simulink model "chap8_5sim"  (Simulink 7.7)
settings: Solver=ode45  StartTime=0.0  StopTime=10  RelTol=1e-3
settings Model: Creator=ljk  LastModifiedBy=ljk  ExtModeTrigMode=oneshot  ExtModeArmWhenConnect=off
settings DataIOCC: LimitDataPoints=off
settings OptimizationCC: BlockReduction=off  BooleanDataType=off
settings DebuggingCC: SaveWithParameterizedLinksMsg=none  SignalResolutionControl=TryResolveAllWithWarning  SolverPrmCheckMsg=none  MultiTaskDSMMsg=warning  MultiTaskCondExecSysMsg=none  StrictBusMsg=None
settings HardwareCC: TargetUnknown=on
settings RTWCC: IncludeERTFirstTime=on

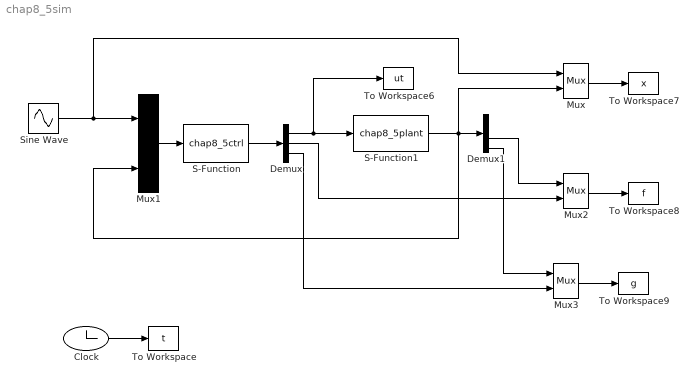
== system chap8_5sim ==
  Clock : Clock
  Demux : Demux  Outputs=3
  Demux1 : Demux
  Mux{,1..3} (4 alike) : Mux  Inputs=2
  S-Function : S-Function  FunctionName=chap8_5ctrl  EnableBusSupport=off
  S-Function1 : S-Function  FunctionName=chap8_5plant  EnableBusSupport=off
  Sine Wave : Sin  Amplitude=0.1  SampleTime=0
  To Workspace : ToWorkspace  VariableName=t  SampleTime=-1  SaveFormat=Array
  To Workspace6 : ToWorkspace  VariableName=ut  SampleTime=-1  SaveFormat=Array
  To Workspace7 : ToWorkspace  VariableName=x  SampleTime=-1  SaveFormat=Array
  To Workspace8 : ToWorkspace  VariableName=f  SampleTime=-1  SaveFormat=Array
  To Workspace9 : ToWorkspace  VariableName=g  SampleTime=-1  SaveFormat=Array
  wires:
  Mux1/1 -> S-Function/1
  S-Function/1 -> Demux/1
  S-Function1/1 -> Demux1/1, Mux/2, Mux1/2
  Sine Wave/1 -> Mux/1, Mux1/1
  Demux/3 -> Mux3/2
  Demux/2 -> Mux2/2
  Demux/1 -> To Workspace6/1, S-Function1/1
  Mux/1 -> To Workspace7/1
  Clock/1 -> To Workspace/1
  Mux2/1 -> To Workspace8/1
  Mux3/1 -> To Workspace9/1
  Demux1/3 -> Mux2/1
  Demux1/4 -> Mux3/1
